simulink model "ServoAmira"  (R2023b)
settings: Solver=ode45  StartTime=0.0  StopTime=5  RelTol=1e-3  EnableMultiTasking=on
InitFcn:
  | g = 9.81; %gravitational constant
  | 
  | 
  | % showVR = 1; %show VR world
  | % ig_init = 0; %initial condition
  | % im_init = 0; %initial condition
  | % omega_init = 0; %initial condition
  | % phi_init = 0; %initial condition
libraries: vrlib x4, simulink x1
CloseFcn:
  | vrclose all;
  | clear figureVR worldVR;
settings Model: Creator=Luky  LastModifiedBy=Lenovo
settings SolverCC: AlgebraicLoopSolver=TrustRegion
settings DataIOCC: LimitDataPoints=on  SaveFormat=Array  SignalLoggingSaveFormat=ModelDataLogs  ReturnWorkspaceOutputs=off
settings OptimizationCC: ExpressionDepthLimit=2147483647  InitFltsAndDblsToZero=on  LifeSpan=inf
settings DebuggingCC: SaveWithParameterizedLinksMsg=none  UnderspecifiedInitializationDetection=Classic  MergeDetectMultiDrivingBlocksExec=none  SolverPrmCheckMsg=warning  FcnCallInpInsideContextMsg=warning  UnconnectedInputMsg=warning  UnconnectedOutputMsg=warning  UnconnectedLineMsg=warning  StateNameClashWarn=warning  SFUnexpectedBacktrackingDiag=warning  SFNoUnconditionalDefaultTransitionDiag=warning  SFExecutionAtInitializationDiag=none  ArithmeticOperatorsInVariantConditions=warning
settings HardwareCC: ProdBitPerPointer=32  ProdBitPerSizeT=32  ProdBitPerPtrDiffT=32  ProdLargestAtomicFloat=None  ProdIntDivRoundTo=Undefined  ProdEndianess=Unspecified  ProdWordSize=32  ProdHWDeviceType=32-bit Generic
settings ModelReferenceCC: PropagateSignalLabelsOutOfModel=off
settings SFSimCC: SimUseLocalCustomCode=off  CustomCodeUndefinedFunction=UseInterfaceOnly
settings RTWCC: RTWUseLocalCustomCode=off
settings CodeAppCC: StateflowObjectComments=on
settings GRTTargetCC: TargetLangStandard=C89/C90 (ANSI)  CombineOutputUpdateFcns=off  GRTInterface=on
settings ConfigComp: CovMetricSettings=dw  CovSaveCumulativeToWorkspaceVar=on  CovSaveSingleToWorkspaceVar=on  CovExternalEMLEnable=off

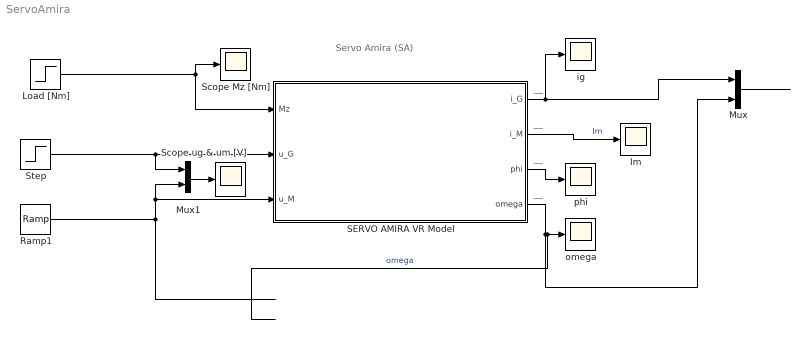
== system ServoAmira ==
  note: Servo Amira (SA)
  note: __
  note: __
  note: __
  note: __
  Im : Scope
  "Load [Nm] " : Step  Time=0  After=0  SampleTime=0
  Mux : Mux  Inputs=2
  Mux1 : Mux  Inputs=2
  Ramp1 : simulink/Sources/Ramp  slope=0  start=0  InitialOutput=0
  SERVO AMIRA VR Model : Subsystem  mask(Servo Amira){showVR=on, sfcnParam1=0, sfcnParam2=0, sfcnParam3=0, sfcnParam4=0}
      mask prompts: showVR "Show VR?"; sfcnParam1 "Initial value of the current of the generator [A]"; sfcnParam2 "Initial value of the current of the motor  im [A]"; sfcnParam3 "Initial value of the angular speed  omega [rad/s]"; sfcnParam4 "Initial value of the angle of the motor shaft phi [rad]"
      mask help: Servo Amira - Virtual Reality
      mask Help:
      | Servo Amira - Virtual Reality <br><br>
      | 
      | 
      | This is a model of the direct current motor. Model is determined to demonstrate real system. It has two inputs, voltage and torgue. Outputs are rotational velocity of the shaft, current and position of the shaft. Virtual reality shows input and output values of the motor.
      | <br><br>
      | 
      | 
      | This is a virtual model of the Servo Amira laboratory model
      | in laboratory of automatic control theory&nbsp;26 (<a href="http://dce.felk.cvut.cz/lab26/" target="_blank">http://dce.felk.cvut.cz/lab26/</a>),
      | which consists of two identical motors (left and right) connected together with a very little flexible shaft. The left motor is used as a generator - it
      | can be used for simulation of a varying  moment of inertia. The right motor is used for control of the rotational speed of the servomechanism or
      | of the angle the motor shaft. <br><br>
      | 
      | There are two inputs and four outputs of the model. The inputs are voltages of the motors um [V] and ug [V] between -10 and 10 volts. Outputs
      | are the speed of the servomechanism omega [rad/s], the angle of the motor shaft phi [rad] and the currents of the motors im [A], ig [A].
      | More information can be found on the website <a href="http://dce.felk.cvut.cz/lab26/" target="_blank">http://dce.felk.cvut.cz/lab26/</a>.<br><br>
      | 
      | 
      | In the mask of the model, it can be set:
      | <ul>
      | <li>Initial value of the current of the generator</li>
      | <li>Initial value of the current of the motor</li>
      | <li>Initial value of the angular speed</li>
      | <li>Initial value of the angle of the motor shaft</li>
      | </ul><br><br>
      | 
      | 
      | Copyright: 2008,   Petr Prochazka, Jirka Roubal, Petr Husek.
      mask Callback showVR:
      | if strcmp('off',get_param(gcb,'showVR'))
      |     vrclose all;
      | else
      |     if exist('figureVR')==0
      |         figureVR = vrfigure;
      |     end
      |     if exist('worldVR')==0
      |         worldVR = vrworld('ServoAmira_VR.WRL');
      |     end
      | 	if isvalid(figureVR)==0
      |         open(worldVR);
      |         figureVR = vrfigure(worldVR,[650 80 550 350]);
      | 	end
      | end
      mask Display:
      | image(imread('ServoAmira_Image.jpg'))
      | port_label ('input',1,'Mz [Nm]')
      | port_label ('input',2,'ug [V]')
      | port_label ('input',3,'um [V]')
      | port_label ('output',1,'ig [A]')
      | port_label ('output',2,'im [A]')
      | port_label ('output',3,'phi [rad]')
      | port_label ('output',4,'omega [rad/s]')
  Scope Mz [Nm] : Scope
  Scope ug & um [V] : Scope
  Step : Step  After=6  SampleTime=0
  ig : Scope
  omega : Scope
  phi : Scope
  wires:
  Step/1 -> Mux1/1, SERVO AMIRA VR Model/2(u_G)
  "Load [Nm] "/1 -> SERVO AMIRA VR Model/1(Mz), Scope Mz [Nm]/1
  Mux1/1 -> Scope ug & um [V]/1
  SERVO AMIRA VR Model/2("i_M ") -> Im/1  "Im"
  SERVO AMIRA VR Model/4("omega ") -> Mux/2, omega/1  "omega"
  Ramp1/1 -> Mux1/2, SERVO AMIRA VR Model/3(u_M)
  SERVO AMIRA VR Model/3("phi ") -> phi/1
  ? -> ?
  SERVO AMIRA VR Model/1(i_G) -> Mux/1, ig/1
  Mux/1 -> ?

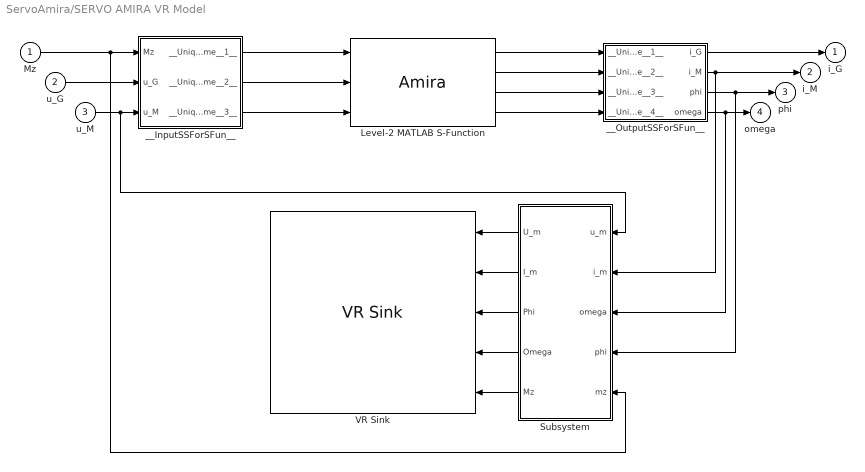
== system ServoAmira/SERVO AMIRA VR Model ==
  Mz : Inport
  u_G : Inport  Port=2
  u_M : Inport  Port=3
  Level-2 MATLAB S-Function : M-S-Function  FunctionName=Amira  Parameters=ig0 im0 omega0 psi0  mask{ig0=sfcnParam1, im0=sfcnParam2, omega0=sfcnParam3, psi0=sfcnParam4}
      mask prompts: ig0 "ig_init"; im0 "im_init"; omega0 "omega_init"; psi0 "psi_init"
      mask Display:
      | port_label('input',1,'Mz');
      | port_label('input',2,'u_G');
      | port_label('input',3,'u_M');
      | port_label('output',1,'i_G');
      | port_label('output',2,'i_M ');
      | port_label('output',3,'phi ');
      | port_label('output',4,'omega ');
  Subsystem : Subsystem
  VR Sink : vrlib/VR Sink  InstantiateOnLoad=on  SampleTime=0.1  ViewEnable=on  RemoteChange=off  RemoteView=on  FieldsWritten=show_u.translation.3.1.double#show_i.translation.3.1.double#fi.rotation.4.1.double#show_n.rotation.4.1.double#show_m.translation.3.1.double  WorldFileName=ServoAmira_VR.WRL  AutoView=off  VideoDimensions=[]  AllowVariableSize=off
  __InputSSForSFun__ : Subsystem
  __OutputSSForSFun__ : Subsystem
  i_G : Outport  OutDataTypeStr=double  PortDimensions=1  SampleTime=[-1 0]
  "i_M " : Outport  Port=2  OutDataTypeStr=double  PortDimensions=1  SampleTime=[-1 0]
  "phi " : Outport  Port=3  OutDataTypeStr=double  PortDimensions=1  SampleTime=[-1 0]
  "omega " : Outport  Port=4  OutDataTypeStr=double  PortDimensions=1  SampleTime=[-1 0]
  wires:
  Mz/1 -> __InputSSForSFun__/1(Mz), Subsystem/5(mz)
  u_G/1 -> __InputSSForSFun__/2(u_G)
  u_M/1 -> __InputSSForSFun__/3(u_M), Subsystem/1(u_m)
  __InputSSForSFun__/1(__UniqueOutportName__1__) -> Level-2 MATLAB S-Function/1
  __InputSSForSFun__/2(__UniqueOutportName__2__) -> Level-2 MATLAB S-Function/2
  __InputSSForSFun__/3(__UniqueOutportName__3__) -> Level-2 MATLAB S-Function/3
  Level-2 MATLAB S-Function/1 -> __OutputSSForSFun__/1(__UniqueInportName__1__)
  Level-2 MATLAB S-Function/2 -> __OutputSSForSFun__/2(__UniqueInportName__2__)
  Level-2 MATLAB S-Function/3 -> __OutputSSForSFun__/3(__UniqueInportName__3__)
  Level-2 MATLAB S-Function/4 -> __OutputSSForSFun__/4(__UniqueInportName__4__)
  __OutputSSForSFun__/1(i_G) -> i_G/1
  __OutputSSForSFun__/2("i_M ") -> "i_M "/1, Subsystem/2(i_m)
  __OutputSSForSFun__/3("phi ") -> "phi "/1, Subsystem/4(phi)
  __OutputSSForSFun__/4("omega ") -> "omega "/1, Subsystem/3(omega)
  Subsystem/1(U_m) -> VR Sink/1
  Subsystem/2(I_m) -> VR Sink/2
  Subsystem/5(Mz) -> VR Sink/5
  Subsystem/3(Phi) -> VR Sink/3
  Subsystem/4(Omega) -> VR Sink/4

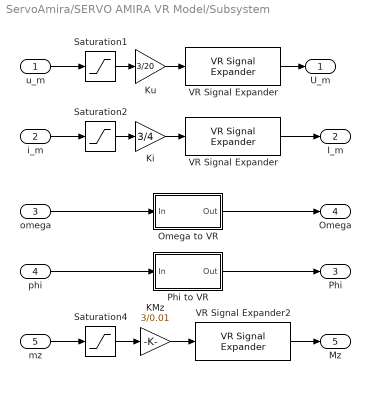
== system ServoAmira/SERVO AMIRA VR Model/Subsystem ==
  u_m : Inport
  i_m : Inport  Port=2
  omega : Inport  Port=3
  phi : Inport  Port=4
  mz : Inport  Port=5
  KMz : Gain  Gain=3/0.01
  Ki : Gain  Gain=3/4
  Ku : Gain  Gain=3/20
  Omega to VR : Subsystem
  Phi to VR : Subsystem
  Saturation1 : Saturate  UpperLimit=10  LowerLimit=-10
  Saturation2 : Saturate  UpperLimit=4  LowerLimit=-4
  Saturation4 : Saturate  UpperLimit=0.005  LowerLimit=-0.005
  VR Signal Expander : vrlib/VR Signal Expander  outwidth=3  outidx=[2]
  "VR Signal Expander " : vrlib/VR Signal Expander  outwidth=3  outidx=[2]
  VR Signal Expander2 : vrlib/VR Signal Expander  outwidth=3  outidx=[2]
  U_m : Outport
  I_m : Outport  Port=2
  Phi : Outport  Port=3
  Omega : Outport  Port=4
  Mz : Outport  Port=5
  wires:
  Ku/1 -> VR Signal Expander/1
  Saturation1/1 -> Ku/1
  Ki/1 -> "VR Signal Expander "/1
  Saturation2/1 -> Ki/1
  Saturation4/1 -> KMz/1
  KMz/1 -> VR Signal Expander2/1
  u_m/1 -> Saturation1/1
  i_m/1 -> Saturation2/1
  phi/1 -> Phi to VR/1(In)
  omega/1 -> Omega to VR/1(In)
  mz/1 -> Saturation4/1
  VR Signal Expander/1 -> U_m/1
  "VR Signal Expander "/1 -> I_m/1
  Phi to VR/1(Out) -> Phi/1
  Omega to VR/1(Out) -> Omega/1
  VR Signal Expander2/1 -> Mz/1

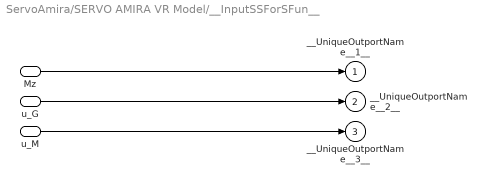
== system ServoAmira/SERVO AMIRA VR Model/__InputSSForSFun__ ==
  Mz : Inport
  u_G : Inport  Port=2
  u_M : Inport  Port=3
  __UniqueOutportName__1__ : Outport
  __UniqueOutportName__2__ : Outport  Port=2
  __UniqueOutportName__3__ : Outport  Port=3
  wires:
  Mz/1 -> __UniqueOutportName__1__/1
  u_G/1 -> __UniqueOutportName__2__/1
  u_M/1 -> __UniqueOutportName__3__/1

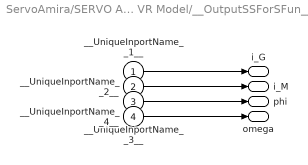
== system ServoAmira/SERVO AMIRA VR Model/__OutputSSForSFun__ ==
  __UniqueInportName__1__ : Inport
  __UniqueInportName__2__ : Inport  Port=2
  __UniqueInportName__3__ : Inport  Port=3
  __UniqueInportName__4__ : Inport  Port=4
  i_G : Outport  OutDataTypeStr=double  PortDimensions=1  SampleTime=[-1 0]
  "i_M " : Outport  Port=2  OutDataTypeStr=double  PortDimensions=1  SampleTime=[-1 0]
  "phi " : Outport  Port=3  OutDataTypeStr=double  PortDimensions=1  SampleTime=[-1 0]
  "omega " : Outport  Port=4  OutDataTypeStr=double  PortDimensions=1  SampleTime=[-1 0]
  wires:
  __UniqueInportName__1__/1 -> i_G/1
  __UniqueInportName__2__/1 -> "i_M "/1
  __UniqueInportName__3__/1 -> "phi "/1
  __UniqueInportName__4__/1 -> "omega "/1

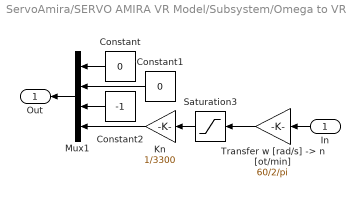
== system ServoAmira/SERVO AMIRA VR Model/Subsystem/Omega to VR ==
  In : Inport
  Constant : Constant  Value=0
  Constant1 : Constant  Value=0
  Constant2 : Constant  Value=-1
  Kn : Gain  Gain=1/3300
  Mux1 : Mux
  Saturation3 : Saturate  UpperLimit=4500  LowerLimit=-4500
  "Transfer w [rad/s] -> n [ot/min]" : Gain  Gain=60/2/pi
  Out : Outport
  wires:
  Constant/1 -> Mux1/1
  Constant1/1 -> Mux1/2
  Constant2/1 -> Mux1/3
  Saturation3/1 -> Kn/1
  Kn/1 -> Mux1/4
  "Transfer w [rad/s] -> n [ot/min]"/1 -> Saturation3/1
  In/1 -> "Transfer w [rad/s] -> n [ot/min]"/1
  Mux1/1 -> Out/1

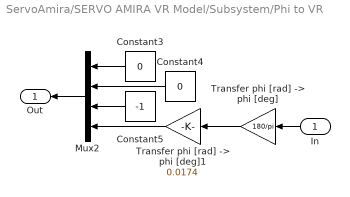
== system ServoAmira/SERVO AMIRA VR Model/Subsystem/Phi to VR ==
  In : Inport
  Constant3 : Constant  Value=0
  Constant4 : Constant  Value=0
  Constant5 : Constant  Value=-1
  Mux2 : Mux
  "Transfer phi [rad] -> phi [deg]" : Gain  Gain=180/pi
  "Transfer phi [rad] -> phi [deg]1" : Gain  Gain=0.0174
  Out : Outport
  wires:
  Constant3/1 -> Mux2/1
  Constant4/1 -> Mux2/2
  Constant5/1 -> Mux2/3
  In/1 -> "Transfer phi [rad] -> phi [deg]"/1
  Mux2/1 -> Out/1
  "Transfer phi [rad] -> phi [deg]"/1 -> "Transfer phi [rad] -> phi [deg]1"/1
  "Transfer phi [rad] -> phi [deg]1"/1 -> Mux2/4
